simulink model "test_qp"  (R2021a)
settings: Solver=VariableStepAuto  StartTime=0.0  StopTime=100.0  RelTol=1e-3
settings Model: Creator=Charles  LastModifiedBy=Charles

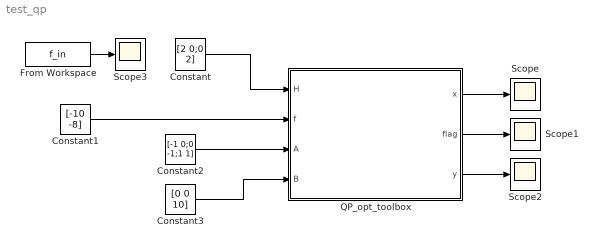
== system test_qp ==
  Constant : Constant  Value=[2 0;0 2]
  Constant1 : Constant  Value=[-10 -8]
  Constant2 : Constant  Value=[-1 0;0 -1;1 1]  VectorParams1D=off
  Constant3 : Constant  Value=[0 0 10]
  From Workspace : FromWorkspace  VariableName=f_in  OutDataTypeStr=single
  QP_opt_toolbox : MATLAB Function  TreatAsAtomicUnit=on
  Scope{,1..3} (4 alike) : Scope
  wires:
  Constant/1 -> QP_opt_toolbox/1(H)
  Constant1/1 -> QP_opt_toolbox/2(f)
  Constant2/1 -> QP_opt_toolbox/3(A)
  Constant3/1 -> QP_opt_toolbox/4(B)
  QP_opt_toolbox/1(x) -> Scope/1
  QP_opt_toolbox/2(flag) -> Scope1/1
  QP_opt_toolbox/3(y) -> Scope2/1
  From Workspace/1 -> Scope3/1

== matlab function test_qp/QP_opt_toolbox ==
  data: x output; flag output; H input; f input; A input; B input; y output
function [x, flag, y] = QP_opt_toolbox(H,f,A,B)  %,varargin
%     x0 = [0.1; 0.3; 0.5; 0; 0.2; 0.3];
    
%     x0 = zeros(size(H, 1), 1);
    x0 = [-1, -2];
    options = optimoptions('quadprog');
    options.Display = 'none';  
    options.Algorithm = 'active-set';
    H = (H + H')/2; % ensure Hessian is symmetric
    [x, y, flag, ~] = quadprog(H, f, A, B, [], [], [], [], x0, options);    %
end
